simulink model "SWC_HALOUT_type"  (R2021b)
settings: Solver=FixedStepDiscrete  StartTime=0.0  StopTime=10.0  FixedStep=0.001  RelTol=1e-3
values from neighbouring files (symbols this model uses):
  DIDLen_APPPedalZP = uint16(3)    [vcu_local_hdr.m]
  DIDLen_APSFunConfig = uint16(16)    [vcu_local_hdr.m]
  DIDLen_AutoLock = uint16(1)    [vcu_local_hdr.m]
  DIDLen_AutoWipHSpdEN = uint16(1)    [vcu_local_hdr.m]
  DIDLen_DKCKey = uint16(8)    [vcu_local_hdr.m]
  DIDLen_DRLDis = uint16(1)    [vcu_local_hdr.m]
  DIDLen_DynoMode = uint16(1)    [vcu_local_hdr.m]
  DIDLen_FMHTimer = uint16(1)    [vcu_local_hdr.m]
  DIDLen_LFLowPresThre = uint16(1)    [vcu_local_hdr.m]
  DIDLen_LFSensorID = uint16(4)    [vcu_local_hdr.m]
  DIDLen_LRLowPresThre = uint16(1)    [vcu_local_hdr.m]
  DIDLen_LRSensorID = uint16(4)    [vcu_local_hdr.m]
  DIDLen_NVMPedalZP = uint16(3)    [vcu_local_hdr.m]
  DIDLen_RFLowPresThre = uint16(1)    [vcu_local_hdr.m]
  DIDLen_RFSensorID = uint16(4)    [vcu_local_hdr.m]
  DIDLen_RRLowPresThre = uint16(1)    [vcu_local_hdr.m]
  DIDLen_RRSensorID = uint16(4)    [vcu_local_hdr.m]
  DIDLen_SensorMode = uint16(1)    [vcu_local_hdr.m]
  DIDLen_TireSize = uint16(16)    [vcu_local_hdr.m]
  DIDLen_TPMSLearnSta = uint16(1)    [vcu_local_hdr.m]
  DIDLen_TurnLampFLThreCurr = uint16(1)    [vcu_local_hdr.m]
  DIDLen_TurnLampFRThreCurr = uint16(1)    [vcu_local_hdr.m]
  DIDLen_TurnLampRLThreCurr = uint16(1)    [vcu_local_hdr.m]
  DIDLen_TurnLampRRThreCurr = uint16(1)    [vcu_local_hdr.m]
  DIDLen_USSConfig = uint16(16)    [vcu_local_hdr.m]
  DIDLen_WhlPres = uint16(4)    [vcu_local_hdr.m]
  DIDLen_WhlSensorBattSta = uint16(1)    [vcu_local_hdr.m]
  DIDLen_WhlTmp = uint16(4)    [vcu_local_hdr.m]
  DIDLen_WipRLSCmdCutFilter = uint16(1)    [vcu_local_hdr.m]
  DIDLen_WipRLSCmdHoldFilter = uint16(1)    [vcu_local_hdr.m]
  DIDLen_XWDMode = uint16(1)    [vcu_local_hdr.m]
  DIDNum_APPPedalZP = uint16(0x0206)    [vcu_local_hdr.m]
  DIDNum_APSFunConfig = uint16(0x0903)    [vcu_local_hdr.m]
  DIDNum_AutoLock = uint16(0x0306)    [vcu_local_hdr.m]
  DIDNum_AutoWipHSpdEN = uint16(0x0308)    [vcu_local_hdr.m]
  DIDNum_DKCKey = uint16(0x0202)    [vcu_local_hdr.m]
  DIDNum_DRLDis = uint16(0x0307)    [vcu_local_hdr.m]
  DIDNum_DynoMode = uint16(0x0203)    [vcu_local_hdr.m]
  DIDNum_FMHTimer = uint16(0x0305)    [vcu_local_hdr.m]
  DIDNum_LFLowPresThre = uint16(0x0B08)    [vcu_local_hdr.m]
  DIDNum_LFSensorID = uint16(0x0B01)    [vcu_local_hdr.m]
  DIDNum_LRLowPresThre = uint16(0x0B0A)    [vcu_local_hdr.m]
  DIDNum_LRSensorID = uint16(0x0B03)    [vcu_local_hdr.m]
  DIDNum_NVMPedalZP = uint16(0x0207)    [vcu_local_hdr.m]
  DIDNum_RFLowPresThre = uint16(0x0B09)    [vcu_local_hdr.m]
  DIDNum_RFSensorID = uint16(0x0B02)    [vcu_local_hdr.m]
  DIDNum_RRLowPresThre = uint16(0x0B0B)    [vcu_local_hdr.m]
  DIDNum_RRSensorID = uint16(0x0B04)    [vcu_local_hdr.m]
  DIDNum_SensorMode = uint16(0x0B0C)    [vcu_local_hdr.m]
  DIDNum_TireSize = uint16(0x0902)    [vcu_local_hdr.m]
  DIDNum_TPMSLearnSta = uint16(0x0B0D)    [vcu_local_hdr.m]
  DIDNum_TurnLampFLThreCurr = uint16(0x0303)    [vcu_local_hdr.m]
  DIDNum_TurnLampFRThreCurr = uint16(0x0301)    [vcu_local_hdr.m]
  DIDNum_TurnLampRLThreCurr = uint16(0x0304)    [vcu_local_hdr.m]
  DIDNum_TurnLampRRThreCurr = uint16(0x0302)    [vcu_local_hdr.m]
  DIDNum_USSConfig = uint16(0x0901)    [vcu_local_hdr.m]
  DIDNum_WhlPres = uint16(0x0B05)    [vcu_local_hdr.m]
  DIDNum_WhlSensorBattSta = uint16(0x0B07)    [vcu_local_hdr.m]
  DIDNum_WhlTmp = uint16(0x0B06)    [vcu_local_hdr.m]
  DIDNum_WipRLSCmdCutFilter = uint16(0x030A)    [vcu_local_hdr.m]
  DIDNum_WipRLSCmdHoldFilter = uint16(0x0309)    [vcu_local_hdr.m]
  DIDNum_XWDMode = uint16(0x0201)    [vcu_local_hdr.m]
  ENUM_TPMSLearnStatus_LEARNED = uint8(  1  )    [vcu_local_hdr.m]
  ENUM_TPMSLearnStatus_LEARNFAIL = uint8(  2  )    [vcu_local_hdr.m]
  ENUM_TPMSLearnStatus_NOTLEARN = uint8(  0  )    [vcu_local_hdr.m]
  FALSE = boolean( 0 )    [vcu_local_hdr.m]    (also in vcu_local_hdrTA2.m)
  TRUE = boolean( 1 )    [vcu_local_hdr.m]    (also in vcu_local_hdrTA2.m)
  ZERO_INT = uint8(0)    [vcu_local_hdr.m]    (also in vcu_local_hdrTA2.m)
undefined symbols (not defined in the file or in its folder): f32_ApsOutVehSpdSig, R_DIDWriteCDD_CSOP_DIDSet_APPPedalZP, R_DIDWriteCDD_CSOP_DIDSet_APSFunConfig, R_DIDWriteCDD_CSOP_DIDSet_AutoLock, R_DIDWriteCDD_CSOP_DIDSet_AutoWipHSpdEN, R_DIDWriteCDD_CSOP_DIDSet_DKCKey, R_DIDWriteCDD_CSOP_DIDSet_DRLDis, R_DIDWriteCDD_CSOP_DIDSet_DynoMode, R_DIDWriteCDD_CSOP_DIDSet_FMHTimer, R_DIDWriteCDD_CSOP_DIDSet_LFLowPresThre, R_DIDWriteCDD_CSOP_DIDSet_LFSensorID, R_DIDWriteCDD_CSOP_DIDSet_LRLowPresThre, R_DIDWriteCDD_CSOP_DIDSet_LRSensorID, R_DIDWriteCDD_CSOP_DIDSet_NVMPedalZP, R_DIDWriteCDD_CSOP_DIDSet_RFLowPresThre, R_DIDWriteCDD_CSOP_DIDSet_RFSensorID, R_DIDWriteCDD_CSOP_DIDSet_RRLowPresThre, R_DIDWriteCDD_CSOP_DIDSet_RRSensorID, R_DIDWriteCDD_CSOP_DIDSet_SensorMode, R_DIDWriteCDD_CSOP_DIDSet_TireSize, R_DIDWriteCDD_CSOP_DIDSet_TPMSLearnSta, R_DIDWriteCDD_CSOP_DIDSet_TurnLampFLThreCurr, R_DIDWriteCDD_CSOP_DIDSet_TurnLampFRThreCurr, R_DIDWriteCDD_CSOP_DIDSet_TurnLampRLThreCurr, R_DIDWriteCDD_CSOP_DIDSet_TurnLampRRThreCurr, R_DIDWriteCDD_CSOP_DIDSet_USSConfig, R_DIDWriteCDD_CSOP_DIDSet_WhlPres, R_DIDWriteCDD_CSOP_DIDSet_WhlSensorBattSta, R_DIDWriteCDD_CSOP_DIDSet_WhlTmp, R_DIDWriteCDD_CSOP_DIDSet_WipRLSCmdCutFilter, R_DIDWriteCDD_CSOP_DIDSet_WipRLSCmdHoldFilter, R_DIDWriteCDD_CSOP_DIDSet_XWDMode, R_FDCCDD_Inner_CSOP_FDC_AppCallSleep, R_HALINCDD_CSOP_PAS_Handler, R_HALINCDD_CSOP_UDS_Main, R_HALOUT_APS_CSOP_ApsOutput, R_HALOUTCDD_CSOP_AppNmStateReq, R_HALOUTCDD_CSOP_ResetPedalZeroPosDone, R_HALOUTCDD_CSOP_SetAcoreRebootCmdACK, R_HALOUTCDD_CSOP_SetHazardIND, R_HALOUTCDD_CSOP_SetSysPwrStat, R_HALOUTCDD_CSOP_SleepRequest, R_HALOUTCDD_CSOP_TPMSSensorIDRegSetResults, R_IOExpOUT_CDD_CSOP_IOExpSetVal, R_J1939_CAN1_FD1_CE100_0_CSOP_Write_CAN1_FD1_CE100_0, R_J1939_CAN1_FD1_CE100_1_CSOP_Write_CAN1_FD1_CE100_1, R_NVMWriteCDD_Inner_NVM_WriteOperation, R_UDSCDD_CSOP_DdmRestartOperationCycle, R_WDGCDD_CSOP_Call_WDG_AppEnd, u16_DIDLen_APPPedalZP, u16_DIDLen_APSFunConfig, u16_DIDLen_AutoLock, u16_DIDLen_AutoWipHSpdEN, u16_DIDLen_DKCKey, u16_DIDLen_DRLDis, u16_DIDLen_DynoMode, u16_DIDLen_FMHTimer, u16_DIDLen_LFLowPresThre, u16_DIDLen_LFSensorID, u16_DIDLen_LRLowPresThre ... (+95)
libraries: FVT_lib x142, simulink x107, hdlsllib x6, hcu_lib x5, halout x1
(part 4 of 8)

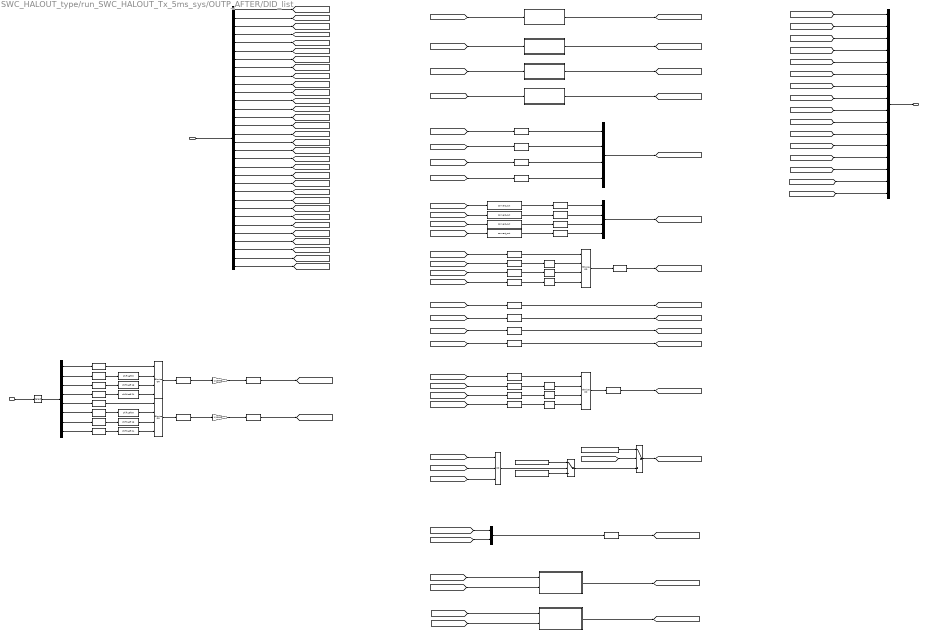
== system SWC_HALOUT_type/run_SWC_HALOUT_Tx_5ms_sys/OUTP_AFTER/DID_list ==
  BOUTP_outputs : Inport
  VHAL_NvmReadArray_raw : Inport  Port=2
  Bit Shift : hdlsllib/Logic and Bit Operations/Bit Shift  mode=Shift Left Logical  N=3
  Bit Shift1 : hdlsllib/Logic and Bit Operations/Bit Shift  mode=Shift Left Logical  N=2
  Bit Shift2 : hdlsllib/Logic and Bit Operations/Bit Shift  mode=Shift Left Logical  N=1
  Bit Shift3 : hdlsllib/Logic and Bit Operations/Bit Shift  mode=Shift Left Logical  N=3
  Bit Shift4 : hdlsllib/Logic and Bit Operations/Bit Shift  mode=Shift Left Logical  N=2
  Bit Shift5 : hdlsllib/Logic and Bit Operations/Bit Shift  mode=Shift Left Logical  N=1
  Bitwise OR : simulink/Logic and Bit Operations/Bitwise Operator  logicop=OR  UseBitMask=off  NumInputPorts=4  BitMask=bin2dec('11011001')  BitMaskRealWorld=Stored Integer
  Bitwise OR1 : simulink/Logic and Bit Operations/Bitwise Operator  logicop=OR  UseBitMask=off  NumInputPorts=4  BitMask=bin2dec('11011001')  BitMaskRealWorld=Stored Integer
  Bitwise OR13 : simulink/Logic and Bit Operations/Bitwise Operator  logicop=OR  UseBitMask=off  NumInputPorts=4  BitMask=bin2dec('00000000000000000000')  BitMaskRealWorld=Stored Integer
  Bitwise OR14 : simulink/Logic and Bit Operations/Bitwise Operator  logicop=OR  UseBitMask=off  NumInputPorts=4  BitMask=bin2dec('00000000000000000000')  BitMaskRealWorld=Stored Integer
  Bus Creator : BusCreator  Inputs=16
  Bus Selector : BusSelector  OutputSignals=VOUTP_WriteChkLFID_raw,VOUTP_WriteChkRFID_raw,VOUTP_WriteChkLRID_raw,VOUTP_WriteChkRRID_raw,VOUTP_LFWheelPress_raw8,VOUTP_RFWheelPress_raw8,VOUTP_LRWheelPress_raw8,VOUTP_RRWheelPress_raw8,VOUTP_LFWheelTemp_C,VOUTP_RFWheelTemp_C,VOUTP_LRWheelTemp_C,VOUTP_RRWheelTemp_C,VOUTP_LFBatWarn_flg,VOUTP_RFBatWarn_flg,VOUTP_LRBatWarn_flg,VOUTP_RRBatWarn_flg,VOUTP_LFWheelPSW_raw8,VOUTP_LRWheelPSW_raw8,VOUTP_RFWheelPSW_raw8,VOUTP_RRWheelPSW_raw8,VOUTP_LFSensorMode_flg,VOUTP_RFSensorMode_flg,VOUTP_LRSensorMode_flg,VOUTP_RRSensorMode_flg,VOUTP_ALFin_flg,VOUTP_ChkStorge_flg,VOUTP_TPMSStorge_flg,VOUTP_unlearnSfali_flg,VOUTP_WritingCnt_enum,VOUTP_LProgress_enum,VOUTP_EAPS1MIN_pct,VOUTP_EAPS2MIN_pct
  Constant : Constant  Value=ENUM_TPMSLearnStatus_LEARNFAIL
  Constant1 : Constant  Value=ENUM_TPMSLearnStatus_NOTLEARN
  Constant2 : Constant  Value=ENUM_TPMSLearnStatus_LEARNED
  Data Type Conversion{1..23} (23 alike) : DataTypeConversion  OutDataTypeStr=uint8
  Data Type Conversion168 : DataTypeConversion  OutDataTypeStr=single
  Data Type Conversion{169..178} (10 alike) : DataTypeConversion  OutDataTypeStr=uint32
  Data Type Conversion179 : DataTypeConversion  OutDataTypeStr=single
  Demux : Demux  Outputs=8
  Logical Operator1 : Logic  Operator=OR  Inputs=3  AllPortsSameDT=off  OutDataTypeStr=boolean
  Multiply1 : Gain  Gain=1/10000
  Multiply2 : Gain  Gain=1/10000
  Mux : Mux
  Mux1 : Mux  Inputs=2
  Mux2 : Mux
  Selector1 : Selector  InputPortWidth=1024  IndexOptions=Index vector (dialog)  Indices=[112:119]  OutputSizes=1
  Shift Arithmetic37 : ArithShift  BitShiftNumber=8  BitShiftDirection=Left
  Shift Arithmetic38 : ArithShift  BitShiftNumber=16  BitShiftDirection=Left
  Shift Arithmetic39 : ArithShift  BitShiftNumber=24  BitShiftDirection=Left
  Shift Arithmetic40 : ArithShift  BitShiftNumber=8  BitShiftDirection=Left
  Shift Arithmetic41 : ArithShift  BitShiftNumber=16  BitShiftDirection=Left
  Shift Arithmetic42 : ArithShift  BitShiftNumber=24  BitShiftDirection=Left
  Switch : Switch  Criteria=u2 ~= 0
  Switch1 : Switch  Criteria=u2 ~= 0
  convert_out{,1..3} (4 alike) : FVT_lib/hal/convert_out  gain=1  offset=-40
  pct2raw1 : Subsystem
  pct2raw8 : Subsystem
  uint32Touint8Array : Subsystem
  uint32Touint8Array1 : Subsystem
  uint32Touint8Array2 : Subsystem
  uint32Touint8Array3 : Subsystem
  BOUTP_DIDSetData_outputs : Outport
  wires:
  BOUTP_outputs/1 -> Bus Selector/1
  Bus Selector/1 -> [VOUTP_WriteChkLFID_raw]  "<VOUTP_WriteChkLFID_raw>"
  Bus Selector/2 -> [VOUTP_WriteChkRFID_raw]  "<VOUTP_WriteChkRFID_raw>"
  Bus Selector/4 -> [VOUTP_WriteChkRRID_raw]  "<VOUTP_WriteChkRRID_raw>"
  Bus Selector/3 -> [VOUTP_WriteChkLRID_raw]  "<VOUTP_WriteChkLRID_raw>"
  Bus Selector/5 -> [VOUTP_LFWheelPress_raw8]  "<VOUTP_LFWheelPress_raw8>"
  Bus Selector/6 -> [VOUTP_RFWheelPress_raw8]  "<VOUTP_RFWheelPress_raw8>"
  Bus Selector/7 -> [VOUTP_LRWheelPress_raw8]  "<VOUTP_LRWheelPress_raw8>"
  Bus Selector/8 -> [VOUTP_RRWheelPress_raw8]  "<VOUTP_RRWheelPress_raw8>"
  Bus Selector/13 -> [VOUTP_LFBatWarn_flg]  "<VOUTP_LFBatWarn_flg>"
  Bus Selector/14 -> [VOUTP_RFBatWarn_flg]  "<VOUTP_RFBatWarn_flg>"
  Bus Selector/15 -> [VOUTP_LRBatWarn_flg]  "<VOUTP_LRBatWarn_flg>"
  Bus Selector/16 -> [VOUTP_RRBatWarn_flg]  "<VOUTP_RRBatWarn_flg>"
  Bus Selector/18 -> [VOUTP_LRWheelPSW_raw8]  "<VOUTP_LRWheelPSW_raw8>"
  Bus Selector/19 -> [VOUTP_RFWheelPSW_raw8]  "<VOUTP_RFWheelPSW_raw8>"
  Bus Selector/20 -> [VOUTP_RRWheelPSW_raw8]  "<VOUTP_RRWheelPSW_raw8>"
  Bus Selector/17 -> [VOUTP_LFWheelPSW_raw8]  "<VOUTP_LFWheelPSW_raw8>"
  Bus Selector/21 -> [VOUTP_LFSensorMode_flg]  "<VOUTP_LFSensorMode_flg>"
  Bus Selector/22 -> [VOUTP_RFSensorMode_flg]  "<VOUTP_RFSensorMode_flg>"
  Bus Selector/23 -> [VOUTP_LRSensorMode_flg]  "<VOUTP_LRSensorMode_flg>"
  Bus Selector/24 -> [VOUTP_RRSensorMode_flg]  "<VOUTP_RRSensorMode_flg>"
  Bus Selector/27 -> [VOUTP_TPMSStorge_flg]  "<VOUTP_TPMSStorge_flg>"
  Bus Selector/25 -> [VOUTP_ALFin_flg]  "<VOUTP_ALFin_flg>"
  Bus Selector/26 -> [VOUTP_ChkStorge_flg]  "<VOUTP_ChkStorge_flg>"
  Bus Selector/28 -> [VOUTP_unlearnSfali_flg]  "<VOUTP_unlearnSfali_flg>"
  Bus Selector/9 -> [VOUTP_LFWheelTemp_C]  "<VOUTP_LFWheelTemp_C>"
  Bus Selector/10 -> [VOUTP_RFWheelTemp_C]  "<VOUTP_RFWheelTemp_C>"
  Bus Selector/11 -> [VOUTP_LRWheelTemp_C]  "<VOUTP_LRWheelTemp_C>"
  Bus Selector/12 -> [VOUTP_RRWheelTemp_C]  "<VOUTP_RRWheelTemp_C>"
  Data Type Conversion8/1 -> Mux2/1
  Data Type Conversion9/1 -> Mux2/2
  Data Type Conversion10/1 -> Mux2/3
  Data Type Conversion11/1 -> Mux2/4
  [VOUTP_LFWheelPSW_raw8] -> Data Type Conversion6/1
  [VOUTP_RRWheelPSW_raw8] -> Data Type Conversion5/1
  [VOUTP_LFSensorMode_flg] -> Data Type Conversion21/1
  [VOUTP_RRSensorMode_flg] -> Data Type Conversion14/1
  [VOUTP_LRSensorMode_flg] -> Data Type Conversion12/1
  [VOUTP_RFSensorMode_flg] -> Data Type Conversion13/1
  Data Type Conversion21/1 -> Bitwise OR/1
  Data Type Conversion12/1 -> Bit Shift1/1
  Data Type Conversion14/1 -> Bit Shift/1
  Constant1/1 -> Switch1/3
  [VOUTP_ALFin_flg] -> Logical Operator1/1
  Switch1/1 -> Switch/3
  [VOUTP_ChkStorge_flg] -> Logical Operator1/2
  Constant/1 -> Switch/1
  Constant2/1 -> Switch1/1
  [VOUTP_TPMSStorge_flg] -> Logical Operator1/3
  Logical Operator1/1 -> Switch1/2
  [VOUTP_unlearnSfali_flg] -> Switch/2
  Mux/1 -> [VHAL_DIDSetWhlPres_raw8]
  Mux2/1 -> [VHAL_DIDSetWhlTmp_raw8]
  Data Type Conversion6/1 -> [VHAL_DIDSetLFLowPresThre_raw8]
  Data Type Conversion7/1 -> [VHAL_DIDSetRFLowPresThre_raw8]
  Data Type Conversion4/1 -> [VHAL_DIDSetLRLowPresThre_raw8]
  Data Type Conversion5/1 -> [VHAL_DIDSetRRLowPresThre_raw8]
  Bitwise OR/1 -> Data Type Conversion20/1
  Switch/1 -> [VHAL_DIDSetTPMSLearnSta_raw8]
  Bit Shift/1 -> Bitwise OR/4
  Bit Shift1/1 -> Bitwise OR/3
  Bit Shift2/1 -> Bitwise OR/2
  Data Type Conversion20/1 -> [VHAL_DIDSetSensorMode_raw8]
  Data Type Conversion13/1 -> Bit Shift2/1
  [VOUTP_RFBatWarn_flg] -> Data Type Conversion2/1
  Data Type Conversion1/1 -> Bit Shift4/1
  [VOUTP_LRBatWarn_flg] -> Data Type Conversion1/1
  [VOUTP_LFBatWarn_flg] -> Data Type Conversion22/1
  Bitwise OR1/1 -> Data Type Conversion15/1
  Bit Shift4/1 -> Bitwise OR1/3
  Data Type Conversion2/1 -> Bit Shift5/1
  Bit Shift3/1 -> Bitwise OR1/4
  Data Type Conversion22/1 -> Bitwise OR1/1
  Data Type Conversion3/1 -> Bit Shift3/1
  Bit Shift5/1 -> Bitwise OR1/2
  [VOUTP_RRBatWarn_flg] -> Data Type Conversion3/1
  Data Type Conversion15/1 -> [VHAL_DIDSetWhlSensorBattSta_raw8]
  [VHAL_DIDSetTPMSLearnSta_raw8] -> Bus Creator/13  "VHAL_DIDSetTPMSLearnSta_raw8"
  [VHAL_DIDSetLFSensorID_raw8] -> Bus Creator/1  "VHAL_DIDSetLFSensorID_raw8"
  [VHAL_DIDSetRFSensorID_raw8] -> Bus Creator/2  "VHAL_DIDSetRFSensorID_raw8"
  [VHAL_DIDSetLRSensorID_raw8] -> Bus Creator/3  "VHAL_DIDSetLRSensorID_raw8"
  [VHAL_DIDSetRRSensorID_raw8] -> Bus Creator/4  "VHAL_DIDSetRRSensorID_raw8"
  [VHAL_DIDSetWhlPres_raw8] -> Bus Creator/5  "VHAL_DIDSetWhlPres_raw8"
  [VHAL_DIDSetWhlTmp_raw8] -> Bus Creator/6  "VHAL_DIDSetWhlTmp_raw8"
  [VHAL_DIDSetWhlSensorBattSta_raw8] -> Bus Creator/7  "VHAL_DIDSetWhlSensorBattSta_raw8"
  [VHAL_DIDSetLFLowPresThre_raw8] -> Bus Creator/8  "VHAL_DIDSetLFLowPresThre_raw8"
  [VHAL_DIDSetRFLowPresThre_raw8] -> Bus Creator/9  "VHAL_DIDSetRFLowPresThre_raw8"
  [VHAL_DIDSetLRLowPresThre_raw8] -> Bus Creator/10  "VHAL_DIDSetLRLowPresThre_raw8"
  [VHAL_DIDSetRRLowPresThre_raw8] -> Bus Creator/11  "VHAL_DIDSetRRLowPresThre_raw8"
  [VHAL_DIDSetSensorMode_raw8] -> Bus Creator/12  "VHAL_DIDSetSensorMode_raw8"
  Bus Creator/1 -> BOUTP_DIDSetData_outputs/1
  [VOUTP_WriteChkLFID_raw] -> uint32Touint8Array/1(In1)
  uint32Touint8Array/1(Out1) -> [VHAL_DIDSetLFSensorID_raw8]
  [VOUTP_WriteChkRFID_raw] -> uint32Touint8Array1/1(In1)
  uint32Touint8Array1/1(Out1) -> [VHAL_DIDSetRFSensorID_raw8]
  [VOUTP_WriteChkLRID_raw] -> uint32Touint8Array2/1(In1)
  uint32Touint8Array2/1(Out1) -> [VHAL_DIDSetLRSensorID_raw8]
  [VOUTP_WriteChkRRID_raw] -> uint32Touint8Array3/1(In1)
  uint32Touint8Array3/1(Out1) -> [VHAL_DIDSetRRSensorID_raw8]
  [VOUTP_RFWheelPress_raw8] -> Data Type Conversion17/1
  [VOUTP_LFWheelPress_raw8] -> Data Type Conversion16/1
  [VOUTP_LRWheelPress_raw8] -> Data Type Conversion18/1
  [VOUTP_RRWheelPress_raw8] -> Data Type Conversion19/1
  convert_out/1 -> Data Type Conversion8/1
  convert_out1/1 -> Data Type Conversion9/1
  convert_out2/1 -> Data Type Conversion10/1
  convert_out3/1 -> Data Type Conversion11/1
  Data Type Conversion16/1 -> Mux/1
  Data Type Conversion17/1 -> Mux/2
  Data Type Conversion18/1 -> Mux/3
  Data Type Conversion19/1 -> Mux/4
  [VOUTP_LFWheelTemp_C] -> convert_out/1
  [VOUTP_RFWheelTemp_C] -> convert_out1/1
  [VOUTP_LRWheelTemp_C] -> convert_out2/1
  [VOUTP_RRWheelTemp_C] -> convert_out3/1
  [VOUTP_RFWheelPSW_raw8] -> Data Type Conversion7/1
  [VOUTP_LRWheelPSW_raw8] -> Data Type Conversion4/1
  Bus Selector/29 -> [VOUTP_WritingCnt_enum]  "<VOUTP_WritingCnt_enum>"
  Bus Selector/30 -> [VOUTP_LProgress_enum]  "<VOUTP_LProgress_enum>"
  [VOUTP_WritingCnt_enum] -> Mux1/2
  [VHAL_TPMSSensorIDRegResults_raw8] -> Bus Creator/14  "VHAL_TPMSSensorIDRegResults_raw8"
  Data Type Conversion23/1 -> [VHAL_TPMSSensorIDRegResults_raw8]
  [VOUTP_LProgress_enum] -> Mux1/1
  Mux1/1 -> Data Type Conversion23/1
  pct2raw8/1(PedalZP_raw8) -> [VHAL_DIDSetAPPPedalZP_raw8]
  pct2raw1/1(PedalZP_raw8) -> [VHAL_DIDSetNVMPedalZP_raw8]
  [VHAL_DIDSetAPPPedalZP_raw8] -> Bus Creator/15  "VHAL_DIDSetAPPPedalZP_raw8"
  [VHAL_DIDSetNVMPedalZP_raw8] -> Bus Creator/16  "VHAL_DIDSetNVMPedalZP_raw8"
  Data Type Conversion174/1 -> Bitwise OR14/1
  Demux/7 -> Data Type Conversion176/1
  Data Type Conversion170/1 -> Shift Arithmetic37/1
  Demux/2 -> Data Type Conversion170/1
  Data Type Conversion168/1 -> [VHAL_EAPS2MINMem_pct]
  Data Type Conversion172/1 -> Shift Arithmetic39/1
  Data Type Conversion169/1 -> Bitwise OR13/1
  Data Type Conversion175/1 -> Shift Arithmetic40/1
  Data Type Conversion176/1 -> Shift Arithmetic41/1
  Data Type Conversion173/1 -> Multiply1/1
  Data Type Conversion177/1 -> Shift Arithmetic42/1
  Data Type Conversion178/1 -> Multiply2/1
  Multiply2/1 -> Data Type Conversion168/1
  Data Type Conversion171/1 -> Shift Arithmetic38/1
  Demux/8 -> Data Type Conversion177/1
  Demux/5 -> Data Type Conversion174/1
  Demux/6 -> Data Type Conversion175/1
  Bitwise OR13/1 -> Data Type Conversion173/1
  Shift Arithmetic41/1 -> Bitwise OR14/3
  Demux/3 -> Data Type Conversion171/1
  Bitwise OR14/1 -> Data Type Conversion178/1
  Shift Arithmetic39/1 -> Bitwise OR13/4
  Multiply1/1 -> Data Type Conversion179/1
  Shift Arithmetic38/1 -> Bitwise OR13/3
  Demux/4 -> Data Type Conversion172/1
  Data Type Conversion179/1 -> [VHAL_EAPS1MINMem_pct]
  Shift Arithmetic42/1 -> Bitwise OR14/4
  Shift Arithmetic40/1 -> Bitwise OR14/2
  Shift Arithmetic37/1 -> Bitwise OR13/2
  Demux/1 -> Data Type Conversion169/1
  Selector1/1 -> Demux/1
  VHAL_NvmReadArray_raw/1 -> Selector1/1
  Bus Selector/31 -> [VOUTP_EAPS1MIN_pct]  "<VOUTP_EAPS1MIN_pct>"
  Bus Selector/32 -> [VOUTP_EAPS2MIN_pct]  "<VOUTP_EAPS2MIN_pct>"
  [VOUTP_EAPS1MIN_pct] -> pct2raw8/1(EAPS1_pct)
  [VOUTP_EAPS2MIN_pct] -> pct2raw8/2(EAPS2_pct)
  [VHAL_EAPS1MINMem_pct] -> pct2raw1/1(EAPS1_pct)
  [VHAL_EAPS2MINMem_pct] -> pct2raw1/2(EAPS2_pct)
